simulink model "ThreeLevel_Ttype_OffGrid_Inverter_Sim"  (R2022b)
settings: Solver=FixedStepAuto  StartTime=0.0  StopTime=1  FixedStep=1e-6  RelTol=1e-3
undefined symbols (not defined in the file): L1
libraries: spsSeriesRLCBranchLib x14, spsMosfetLib x12, spsRMSLib x10, slpidlib x5, simulink x3, spsThreePhaseVIMeasurementLib x3, spsVoltageMeasurementLib x3, spsDCVoltageSourceLib x1, spsGroundLib x1, spsPower3phInstantaneousLib x1, sps_lib x1
(part 2 of 2)

== matlab function ThreeLevel_Ttype_OffGrid_Inverter_Sim/adc转dq2 ==
  data: a input; b input; c input; d output; theta input; q output
function [d, q] = abc_to_dq_90deg(a, b, c, theta)
% ######################################################################
% 3输入 (a, b, c, theta) -> 2输出 (d, q) 的分立式坐标变换
% 严格匹配 Simulink 模式: 90 degrees behind phase A axis
% ######################################################################

    % ----------- 1. 分立式克拉克变换 (abc -> alpha/beta) -----------
    % 采用等幅值标准系数
    alpha = (2.0 / 3.0) * a - (1.0 / 3.0) * b - (1.0 / 3.0) * c;
    beta  = (1.0 / sqrt(3.0)) * b - (1.0 / sqrt(3.0)) * c;

    % ----------- 2. 三角函数计算 -----------
    cos_theta = cos(theta);
    sin_theta = sin(theta);

    % ----------- 3. 修正后的帕克变换 (匹配 90 deg behind 逻辑) -----------
    % 注意：这里的正负号和三角函数组合与 0 度对齐不同
    d =  alpha * sin_theta - beta * cos_theta;
    q =  alpha * cos_theta + beta * sin_theta;

end

== matlab function ThreeLevel_Ttype_OffGrid_Inverter_Sim/MATLAB Function ==
  data: tsa input; U1 output; tsb input; tsc input; V1 output; W1 output; U2 output; V2 output; W2 output; V_offset_scope output
function [U1, V1, W1, U2, V2, W2, V_offset_scope] = fcn(tsa, tsb, tsc)
%#codegen
% =========================================================================
% 功能: 简化版载波等效三电平SVPWM算法（含三次谐波可视化输出端口）
% 输入: tsa, tsb, tsc —— 三相标准正弦波信号（幅值代表调制比 m）
% 输出: 
%   U1, V1, W1: 范围在 -8500 ~ 8500 的标准基准调制波
%   U2, V2, W2: 范围在 0 ~ 17000 的抬升调制波
%   V_offset_scope: 缩放到定时器计数域的三次谐波波形 (范围约 +/-1700)
% =========================================================================

%% 1. 定义系统常数与硬件计数周期
ARR = 8500; % 半个开关周期计数值（对应单三角载波峰值）

% k 为调制比缩放系数，此处使用你代码中提供的 1.1547 (2/sqrt(3))
% 注意：使用该系数且输入幅值为 0.7542 时，最终物理线电压有效值为 32VRMS。
k = 1/0.866;  

%% 2. 基准缩放 (对应图中的 K- 模块)
va = k * tsa;
vb = k * tsb;
vc = k * tsc;

%% 3. 逻辑归一化（对应图中 Switch 模块逻辑）
if va > 0
    ya = va;
else
    ya = va + 1.0;
end

if vb > 0
    yb = vb;
else
    yb = vb + 1.0;
end

if vc > 0
    yc = vc;
else
    yc = vc + 1.0;
end

%% 4. 寻找虚拟空间的最值
y_max = max([ya, yb, yc]);
y_min = min([ya, yb, yc]);

%% 5. 三次谐波/零序分量注入计算 (Normalized)
v_offset = 0.5 * (1.0 - y_max - y_min);

%% 6. 合成基础归一化羊角波（此时范围严格在 [-1, 1] 空间内）
sa_norm = va + v_offset;
sb_norm = vb + v_offset;
sc_norm = vc + v_offset;

%% 7. 硬件计数域缩放与双波复制
% 放大到定时器半周期计数值域 [-8500, 8500]
U1 = sa_norm * double(ARR);
V1 = sb_norm * double(ARR);
W1 = sc_norm * double(ARR);

% 整体向上抬升一个 ARR，范围变为 [0, 17000]
U2 = U1 + double(ARR);
V2 = V1 + double(ARR);
W2 = W1 + double(ARR);

%% 8. 【新增】将三次谐波波形也放大到硬件计数域，用于在 Scope 中清晰观察
V_offset_scope = v_offset * double(ARR);

end
